simulink library "lib_dGrid"  (R2023b)
settings: Solver=VariableStepAuto  StartTime=0.0  StopTime=10.0  RelTol=1e-3
values from neighbouring files (symbols this model uses):
  C_PM = 10e-3    (= 0.01)    [my_MMC_param.m]
  Cbase = 1/Zbase/wb    (= 3.10849498226e-05)    [my_MMC_param.m]
  f0 = 50/fb    (= 1)    [my_MMC_param.m]
  Fn_filter = 1000    [my_MMC_param.m]
  Fnom = 50    [my_MMC_param.m]
  GFL_APC = 1    [Analysis_Main.m]    (also in initSimu.m; my_MMC_param.m)
  GFL_DVC = 2    [Analysis_Main.m]    (also in initSimu.m; my_MMC_param.m)
  GFM_APC = 3; (values programmed in EMT models)    [Analysis_Main.m]    (also in initSimu.m; my_MMC_param.m = 3)
  GFM_VF = 0    [my_MMC_param.m]
  Ibase = 2*Sbase/(3*Ubase)    [my_MMC_param.m]
  Idcb = Sbase/Udcb    [my_MMC_param.m]
  Ki_Iccsc = 5.15    [my_MMC_param.m]
  Ki_Ireg = CCCTRL.CC.ki    [my_MMC_param.m]
  Ki_Izscc = 100    [my_MMC_param.m]
  Ki_PLL = 1/(CCCTRL.PLL.v0*CCCTRL.PLL.T^2)    [my_MMC_param.m]
  Ki_Preg = 1.0*10    (= 10)    [my_MMC_param.m]
  Ki_Qreg = 1.0*10    (= 10)    [my_MMC_param.m]
  Ki_VAC_GFL = 50    [my_MMC_param.m]
  Ki_VACreg = 10    [my_MMC_param.m]
  Ki_VDCreg = 10    [my_MMC_param.m]
  Ki_WtReg = Kp_WtReg / 0.025    (= 1600)    [my_MMC_param.m]
  Kp_Iccsc = 0.21    [my_MMC_param.m]
  Kp_Ireg = CCCTRL.CC.kp    [my_MMC_param.m]
  Kp_Izscc = 10    [my_MMC_param.m]
  Kp_PLL = 2/CCCTRL.PLL.v0/CCCTRL.PLL.T    [my_MMC_param.m]
  Kp_Preg = 0.5/3*1    (= 0.166666666667)    [my_MMC_param.m]
  Kp_Qreg = 0.5/3*1    (= 0.166666666667)    [my_MMC_param.m]
  Kp_VAC_GFL = 0.5    [my_MMC_param.m]
  Kp_VACreg = 0.01    [my_MMC_param.m]
  Kp_VDCreg = 1    [my_MMC_param.m]
  Kp_WtReg = 40    [my_MMC_param.m]
  Kpv_GFM = 1    [my_MMC_param.m]
  Kpwm = 0.5    [my_MMC_param.m]
  Larm = Larm_pu*(Zbase/wb)    (= 0.0488923985178)    [my_MMC_param.m]
  Lff = Larm_pu/2    (= 0.075)    [my_MMC_param.m]
  Limits_Ireg = [ 2.0  -2.0]    [my_MMC_param.m]
  Limits_Preg = [ 2, -2 ]    [my_MMC_param.m]
  Limits_Qreg = 2*[ 0.42, -0.42 ]    [my_MMC_param.m]
  Limits_VACreg = [ 1.3  -1.3]    [my_MMC_param.m]
  Limits_VDCreg = [ 2.0  -2.0]    [my_MMC_param.m]
  MMC1 = MMC    [Analysis_Main.m]    (also in initSimu.m)
  Nb_PM = 400    [my_MMC_param.m]
  PhaseDelay = 1.0*Ts_Control*2*pi*50    (= 0.0628318530718)    [my_MMC_param.m]
  Pnom = 1000e6    (= 1000000000)    [my_MMC_param.m]
  Rarm = Rarm_pu*Zbase    (= 0.1536)    [my_MMC_param.m]
  Slope_Pref = 0.5    [my_MMC_param.m]
  Slope_Qref = 0.5    [my_MMC_param.m]
  Slope_Vdc_ref = Vnom_dc/2    (= 320000)    [my_MMC_param.m]
  Tdeblock = 1.5    [my_MMC_param.m]
  Ton_CROSSreg = Ton_PQreg+3    (= 7)    [my_MMC_param.m]
  Ton_PQreg = 4    [my_MMC_param.m]
  Ton_VDCreg = 1.5    [my_MMC_param.m]
  Ts = Ts_Control    (= 0.0002)    [my_MMC_param.m]
  Ts_Control = Ts_Power*2    (= 0.0002)    [my_MMC_param.m]
  Ts_Power = 20e-6 * 5    (= 0.0001)    [my_MMC_param.m]
  Ubase = sqrt(2/3)*Vnom_sec    [my_MMC_param.m]
  Udcb = 2*Ubase    [my_MMC_param.m]
  Vc0_PM = 0    [my_MMC_param.m]
  Vnom_dc = 640e3    (= 640000)    [my_MMC_param.m]
  Vnom_sec = 320e3    (= 320000)    [my_MMC_param.m]
  wb = 2*pi*fb    (= 314.159265359)    [my_MMC_param.m]
  Wt_ref_pu = 0.5 * C_PM * (Vnom_dc/Nb_PM)^2 * Nb_PM * 6 / Pnom    (= 0.03072)    [my_MMC_param.m]
undefined symbols (not defined in the file or in its folder): ControlSampleTime, DiscIntNeverNeededParam, MMC, PLL, VSM
libraries: simulink x50, spsCurrentMeasurementLib x20, spsSecondOrderFilterLib x20, spsDiodeLib x12, spsControlledVoltageSourceLib x12, spsSeriesRLCBranchLib x10, spsFirstOrderFilterLib x9, spsVoltageMeasurementLib x8, spsMeanLib x7, FriedrichLibrary x6, $bdroot x6, powerlib_extras x4
(part 4 of 8)

== system lib_dGrid/MMC-configurable control modes/MMC Control/VSM Control ==
  IdIq : Inport  PortDimensions=2
  VdVq : Inport  Port=2  PortDimensions=2
  Pref : Inport  Port=3  PortDimensions=1
  Qref : Inport  Port=4  PortDimensions=1
  wt_PLL : Inport  Port=5  PortDimensions=1
  Pmeas : Inport  Port=6
  Qmeas : Inport  Port=7
  Enable : EnablePort  StatesWhenEnabling=reset
  Add : Sum  Inputs=-++
  Bus Selector1 : BusSelector  OutputSignals=enable,Param.VSM,sp_VSM
  Constant : Constant  Value=1.12
  Constant1 : Constant  Value=[0 0]
  DQ damping1 Need New paras or New implementation : Subsystem  Commented=on  mask(Lead Lag){OmLead=VSM.VTFF.OmLead, OmLag=VSM.VTFF.OmLag}
      mask prompts: OmLead "Omega Lead"; OmLag "Omega Lag"
  Gain : Gain  Commented=on  Gain=0
  Gain4 : Gain  Gain=[1 0]
  Gain7 : Gain  Gain=Ctrl.IsVIinGFM
  Inner Loop Control : Subsystem
  Inner loop flag : Constant  Value=Ctrl.IsCCinGFM
  Modulation Gain : Subsystem  Commented=through
  Mux3 : Mux  Inputs=2
  Saturation : Saturate  Commented=through  UpperLimit=Limits_Ireg(1)  LowerLimit=Limits_Ireg(2)
  Second-Order Filter2 : spsSecondOrderFilterLib/Second-Order Filter  Commented=through  FilterType=Lowpass  Fo=Fn_filter  Zeta=Zeta_filter  Ts=Ts  Initialize=off  Vac_Init="[0,  0,  60]"  Vdc_Init=0  PlotResponse=off  FreqRange=[0, 500, 1]
      settings: LibrarySourceBlock=|
      | sps_lib/Control/Filters/Second-Order
      | Filter
  Should it be a coeffecient in the left block? : Gain  Commented=through  Gain=0.5
  Step : Step  Commented=on  Time=5  SampleTime=Ts_Control
  Switch2 : Switch  Criteria=u2 > Threshold  Threshold=0.5  SaturateOnIntegerOverflow=off  InputSameDT=off
  Unit Delay : UnitDelay  SampleTime=Ts_Control  HasFrameUpgradeWarning=on
  VSM1 : Subsystem
  Virtual circuit daniel style1 : Subsystem
  cmd_VSM : Subsystem
  Uref_dq : Outport  VectorParamsAs1DForOutWhenUnconnected=off
  Phi [rad] : Outport  Port=2  VectorParamsAs1DForOutWhenUnconnected=off
  meas_theta_GFM : Outport  Port=3  VectorParamsAs1DForOutWhenUnconnected=off
  wires:
  Should it be a coeffecient in the left block?/1 -> Saturation/1
  Modulation Gain/1(out) -> Should it be a coeffecient in the left block?/1
  VSM1/1(E [pu]) -> Gain4/1
  Gain4/1 -> Add/2
  Constant/1 -> VSM1/5(init E [pu])
  wt_PLL/1 -> VSM1/4(init Phi [rad])
  cmd_VSM/1(cmd_ac) -> Bus Selector1/1
  Bus Selector1/3 -> VSM1/2(sp_VSM)  "<sp_VSM>"
  Bus Selector1/1 -> Unit Delay/1  "<enable>"
  Bus Selector1/2 -> VSM1/1(Param)  "<VSM>"
  Unit Delay/1 -> VSM1/Enable
  Mux3/1 -> VSM1/3(PQ_meas[pu])
  Step/1 -> DQ damping1 Need New paras or New implementation/1(enable_damp_dq)
  VdVq/1 -> DQ damping1 Need New paras or New implementation/2(u_dq0), Second-Order Filter2/1
  Constant1/1 -> Add/3
  Virtual circuit daniel style1/1(v_vc_dq) -> Gain7/1
  Gain7/1 -> Add/1
  Saturation/1 -> Uref_dq/1
  IdIq/1 -> Virtual circuit daniel style1/1(i_dq), Inner Loop Control/1(IdIq)
  DQ damping1 Need New paras or New implementation/1(damp_dq0) -> Gain/1
  Second-Order Filter2/1 -> Inner Loop Control/3(VdVq)
  Inner Loop Control/1(Out) -> Switch2/1
  Add/1 -> Switch2/3, Inner Loop Control/2(In)
  Switch2/1 -> Modulation Gain/1(Uref)
  Inner loop flag/1 -> Switch2/2, Inner Loop Control/Enable
  Pmeas/1 -> Mux3/1
  Qmeas/1 -> Mux3/2
  Pref/1 -> cmd_VSM/1(Pref)  "2"
  Qref/1 -> cmd_VSM/2(Qref)  "2"
  VSM1/3(meas_theta_GFM) -> meas_theta_GFM/1
  VSM1/2(wt_VSM) -> Phi [rad]/1

== system lib_dGrid/MMC-configurable control modes/MMC Control/u//l arms to ac//dc ==
  In1 : Inport
  In2 : Inport  Port=2
  In3 : Inport  Port=3
  In4 : Inport  Port=4
  Gain2 : Gain  Gain=1/2
  I->pu (Ibase instead of Idcb) : Gain  Gain=1/Ibase  SaturateOnIntegerOverflow=on  OutDataTypeStr=Inherit: Same as input  ParamDataTypeStr=Inherit: Same as input
  Plus1 : Sum  Inputs=+-
  Plus2 : Sum
  Plus3 : Sum
  V->pu1 : Gain  Gain=Nb_PM/Ubase  SaturateOnIntegerOverflow=on  OutDataTypeStr=Inherit: Same as input  ParamDataTypeStr=Inherit: Same as input
  V->pu2 : Gain  Gain=Nb_PM/Ubase  SaturateOnIntegerOverflow=on  OutDataTypeStr=Inherit: Same as input  ParamDataTypeStr=Inherit: Same as input
  Out1 : Outport
  Out2 : Outport  Port=2
  Out3 : Outport  Port=3
  wires:
  Gain2/1 -> I->pu (Ibase instead of Idcb)/1
  Plus3/1 -> V->pu1/1
  Plus2/1 -> Gain2/1
  In2/1 -> Plus3/1, Plus1/2
  In1/1 -> Plus3/2, Plus1/1
  Plus1/1 -> V->pu2/1
  In3/1 -> Plus2/1
  I->pu (Ibase instead of Idcb)/1 -> Out3/1
  In4/1 -> Plus2/2
  V->pu1/1 -> Out1/1
  V->pu2/1 -> Out2/1

== system lib_dGrid/TL-VSC-configurable control modes/VSC Control/APC & Q//Vac Regulator ==
  note: Reactive Power Regulator
  note: Active Power Regulator
  Pmeas : Inport  PortDimensions=1
  Pref : Inport  Port=2  PortDimensions=1  SampleTime=Ts
  Qmes : Inport  Port=3  PortDimensions=1
  Qref : Inport  Port=4  PortDimensions=1
  VdVq_mes : Inport  Port=5  PortDimensions=2
  Enable : EnablePort  StatesWhenEnabling=reset
  Constant : Constant  Value=Ctrl.IsVacGFL
  Discrete-Time Integrator : DiscreteIntegrator  SampleTime=Ts  LimitOutput=on  UpperSaturationLimit=Limits_Qreg(1)  LowerSaturationLimit=Limits_Qreg(2)  ICPrevOutput=DiscIntNeverNeededParam  ICPrevScaledInput=DiscIntNeverNeededParam
  Discrete-Time Integrator1 : DiscreteIntegrator  SampleTime=Ts  LimitOutput=on  UpperSaturationLimit=Limits_Preg(1)  LowerSaturationLimit=Limits_Preg(2)  ICPrevOutput=DiscIntNeverNeededParam  ICPrevScaledInput=DiscIntNeverNeededParam
  Product{,1..3} (4 alike) : Product  RndMeth=Zero
  Rtot_pu1 : Gain  Gain=-1  SaturateOnIntegerOverflow=on  OutDataTypeStr=Inherit: Same as input  ParamDataTypeStr=Inherit: Same as input
  Saturation1 : Saturate  UpperLimit=Limits_Preg(1)  LowerLimit=Limits_Preg(2)  SampleTime=Ts
  Saturation2 : Saturate  UpperLimit=Limits_Qreg(1)  LowerLimit=Limits_Qreg(2)
  Sum : Sum  Inputs=|-+
  Sum1 : Sum  Inputs=|-+
  Sum2 : Sum  InputSameDT=on  SaturateOnIntegerOverflow=on  SampleTime=Ts  OutDataTypeStr=Inherit: Same as first input
  Sum6 : Sum  InputSameDT=on  SaturateOnIntegerOverflow=on  SampleTime=Ts  OutDataTypeStr=Inherit: Same as first input
  Switch3 : Switch  Criteria=u2 > Threshold  Threshold=0.5  OutDataTypeStr=double  SaturateOnIntegerOverflow=off  InputSameDT=off
  VAC control : Subsystem
  VdcNom_SM : Constant  Value=Kp_Qreg
  VdcNom_SM1 : Constant  Value=Ki_Qreg
  VdcNom_SM2 : Constant  Value=Kp_Preg  SampleTime=Ts
  VdcNom_SM3 : Constant  Value=Ki_Preg  SampleTime=Ts
  Zero-Order Hold : ZeroOrderHold  Commented=through  SampleTime=Ts
  Zero-Order Hold1 : ZeroOrderHold  Commented=through  SampleTime=Ts
  Id_ref_Pctrl : Outport  SampleTime=Ts  VectorParamsAs1DForOutWhenUnconnected=off
  Iq_ref : Outport  Port=2  VectorParamsAs1DForOutWhenUnconnected=off
  wires:
  Saturation2/1 -> Rtot_pu1/1
  Switch3/1 -> Iq_ref/1
  Sum6/1 -> Saturation2/1
  Sum/1 -> Product1/2, Product/2
  Product/1 -> Discrete-Time Integrator/1
  Product1/1 -> Zero-Order Hold/1
  VdcNom_SM/1 -> Product1/1
  VdcNom_SM1/1 -> Product/1
  Discrete-Time Integrator/1 -> Sum6/2
  Zero-Order Hold/1 -> Sum6/1
  Qref/1 -> Sum/2
  Rtot_pu1/1 -> Switch3/3
  Constant/1 -> Switch3/2, VAC control/Enable
  VdVq_mes/1 -> VAC control/1(Vdq_meas)
  VAC control/1(Out1) -> Switch3/1
  VdcNom_SM3/1 -> Product2/1
  Product3/1 -> Zero-Order Hold1/1
  Pmeas/1 -> Sum1/1
  Discrete-Time Integrator1/1 -> Sum2/2
  Zero-Order Hold1/1 -> Sum2/1
  Product2/1 -> Discrete-Time Integrator1/1
  Sum1/1 -> Product3/2, Product2/2
  Pref/1 -> Sum1/2
  Saturation1/1 -> Id_ref_Pctrl/1
  VdcNom_SM2/1 -> Product3/1
  Sum2/1 -> Saturation1/1
  Qmes/1 -> Sum/1

== system lib_dGrid/TL-VSC-configurable control modes/VSC Control/Classic//Cross GFL ->Id* ==
  Id_P : Inport
  PQreg_On : Inport  Port=2
  Id_Udc : Inport  Port=3
  Iq_ref : Inport  Port=4
  Mux : Mux  Inputs=2
  Switch4 : Switch  Criteria=u2 ~= 0  Threshold=0.5  OutDataTypeStr=double  SaturateOnIntegerOverflow=off  InputSameDT=off
  Out1 : Outport
  Out2 : Outport  Port=2
  wires:
  Id_P/1 -> Switch4/1
  PQreg_On/1 -> Switch4/2
  Mux/1 -> Out2/1
  Iq_ref/1 -> Mux/2
  Switch4/1 -> Mux/1, Out1/1
  Id_Udc/1 -> Switch4/3

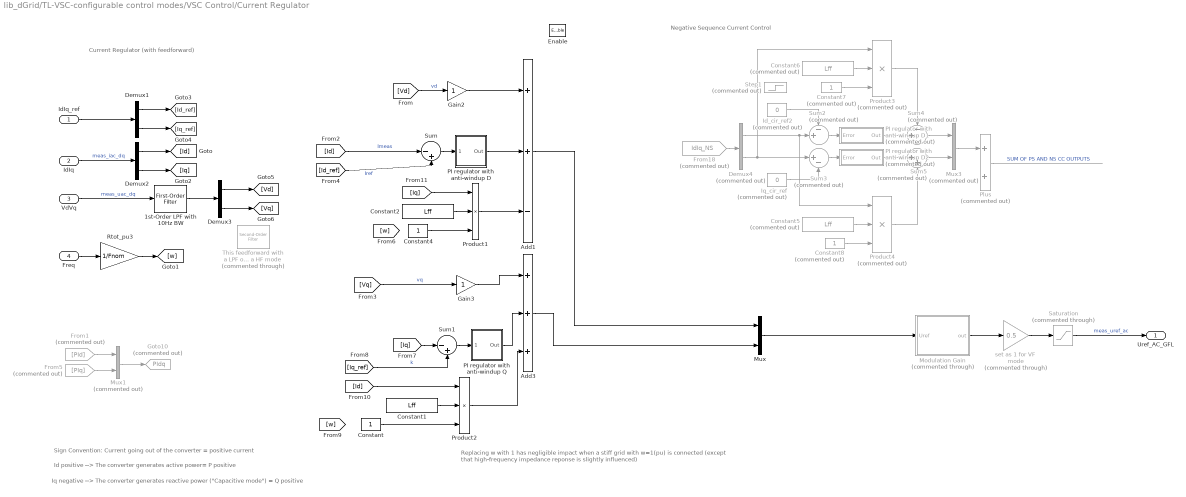
== system lib_dGrid/TL-VSC-configurable control modes/VSC Control/Current Regulator ==
  note: Negative Sequence Current Control
  note: Id positive --> The converter generates active power= P positive
  note: Iq negative --> The converter generates reactive power ("Capacitive mode") = Q positive
  note: Sign Convention: Current going out of the converter = positive current
  note: Current Regulator
      | (with feedforward)
  note: Replacing w with 1 has negligible impact
      | when a stiff grid with w=1(pu) is connected (except that high-frequency impedance reponse is slightly influenced)
  IdIq_ref : Inport  PortDimensions=2
  IdIq : Inport  Port=2  PortDimensions=2
  VdVq : Inport  Port=3  PortDimensions=2
  Freq : Inport  Port=4  PortDimensions=1
  Enable : EnablePort  StatesWhenEnabling=reset
  1st-Order LPF with 10Hz BW : spsFirstOrderFilterLib/First-Order Filter  FilterType=Lowpass  Tc=1/(2*pi*Fn_filter/100)  Ts=Ts  Initialize=off  Vac_Init=[0, 0, 50]  Vdc_Init=0  PlotResponse=off  FreqRange="[0,  200,  1]"
  Add1 : Sum  Inputs=++-
  Add3 : Sum  Inputs=+++
  Constant : Constant
  Constant1 : Constant  Value=Lff  SampleTime=Ts_Control
  Constant2 : Constant  Value=Lff  SampleTime=Ts_Control
  Constant4 : Constant
  Constant5 : Constant  Commented=on  Value=Lff  SampleTime=Ts_Control
  Constant6 : Constant  Commented=on  Value=Lff  SampleTime=Ts_Control
  Constant7 : Constant  Commented=on
  Constant8 : Constant  Commented=on
  Demux1 : Demux  Outputs=2
  Demux2 : Demux  Outputs=2
  Demux3 : Demux  Outputs=2
  Demux4 : Demux  Commented=on  Outputs=2
  From1 : From  Commented=on  GotoTag=PId
  From18 : From  Commented=on  GotoTag=IdIq_NS
  From5 : From  Commented=on  GotoTag=PIq
  Gain2 : Gain
  Gain3 : Gain
  Goto10 : Goto  Commented=on  GotoTag=PIdq  TagVisibility=global
  Id_cir_ref2 : Constant  Commented=on  Value=0
  Iq_cir_ref : Constant  Commented=on  Value=0
  Modulation Gain : Subsystem  Commented=through
  Mux : Mux  Inputs=2
  Mux1 : Mux  Commented=on  Inputs=2
  Mux3 : Mux  Commented=on  Inputs=2
  PI regulator with anti-windup D : Subsystem  DialogController=POWERSYS.PowerSysDialog  mask(Discrete PI Controller){Kp=Kp_Ireg, Ki=Ki_Ireg, Par_Limits=Limits_Ireg, Init=0, Ts=Ts}
      mask prompts: Kp "Proportional gain (Kp):"; Ki "Integral gain (Ki):"; Par_Limits "Output limits: [ Upper   Lower ]"; Init "Output initial value:"; Ts "Sample time:"
      mask help: This block implements a discrete PI controller.
      mask init:
      | UpperLimit=Par_Limits(1);
      | LowerLimit=Par_Limits(2);
      | power_initmask();
      mask Help: This block is part of a subset of blocks in the Extras library that does not have documentation associated with it, other than the block mask description.
      mask Display: disp('PI');
  PI regulator with anti-windup D1 : Subsystem  Commented=on  DialogController=POWERSYS.PowerSysDialog  mask(Discrete PI Controller){Kp=Kp_Ireg, Ki=Ki_Ireg, Par_Limits=Limits_Ireg, Init=0, Ts=Ts}
      mask prompts: Kp "Proportional gain (Kp):"; Ki "Integral gain (Ki):"; Par_Limits "Output limits: [ Upper   Lower ]"; Init "Output initial value:"; Ts "Sample time:"
      mask help: This block implements a discrete PI controller.
      mask init:
      | UpperLimit=Par_Limits(1);
      | LowerLimit=Par_Limits(2);
      | power_initmask();
      mask Help: This block is part of a subset of blocks in the Extras library that does not have documentation associated with it, other than the block mask description.
      mask Display: disp('PI');
  PI regulator with anti-windup D2 : Subsystem  Commented=on  DialogController=POWERSYS.PowerSysDialog  mask(Discrete PI Controller){Kp=Kp_Ireg, Ki=Ki_Ireg, Par_Limits=Limits_Ireg, Init=0, Ts=Ts}
      mask prompts: Kp "Proportional gain (Kp):"; Ki "Integral gain (Ki):"; Par_Limits "Output limits: [ Upper   Lower ]"; Init "Output initial value:"; Ts "Sample time:"
      mask help: This block implements a discrete PI controller.
      mask init:
      | UpperLimit=Par_Limits(1);
      | LowerLimit=Par_Limits(2);
      | power_initmask();
      mask Help: This block is part of a subset of blocks in the Extras library that does not have documentation associated with it, other than the block mask description.
      mask Display: disp('PI');
  PI regulator with anti-windup Q : Subsystem  DialogController=POWERSYS.PowerSysDialog  mask(Discrete PI Controller){Kp=Kp_Ireg, Ki=Ki_Ireg, Par_Limits=Limits_Ireg, Init=0, Ts=Ts}
      mask prompts: Kp "Proportional gain (Kp):"; Ki "Integral gain (Ki):"; Par_Limits "Output limits: [ Upper   Lower ]"; Init "Output initial value:"; Ts "Sample time:"
      mask help: This block implements a discrete PI controller.
      mask init:
      | UpperLimit=Par_Limits(1);
      | LowerLimit=Par_Limits(2);
      | power_initmask();
      mask Help: This block is part of a subset of blocks in the Extras library that does not have documentation associated with it, other than the block mask description.
      mask Display: disp('PI');
  Plus : Sum  Commented=on
  Product1 : Product  Inputs=3  RndMeth=Zero
  Product2 : Product  Inputs=3  RndMeth=Zero
  Product3 : Product  Commented=on  Inputs=3  RndMeth=Zero
  Product4 : Product  Commented=on  Inputs=3  RndMeth=Zero
  Rtot_pu3 : Gain  Gain=1/Fnom  SaturateOnIntegerOverflow=on  OutDataTypeStr=Inherit: Same as input  ParamDataTypeStr=Inherit: Same as input
  Saturation : Saturate  Commented=through  UpperLimit=Limits_Ireg(1)  LowerLimit=Limits_Ireg(2)
  Step1 : Step  Commented=on  Time=10  After=0.02  SampleTime=0
  Sum : Sum  Inputs=|-+
  Sum1 : Sum  Inputs=|-+
  Sum2 : Sum  Commented=on  Inputs=-+|
  Sum3 : Sum  Commented=on  Inputs=|+-
  Sum4 : Sum  Commented=on  Inputs=-+|
  Sum5 : Sum  Commented=on  Inputs=|++
  This feedforward with a LPF of 1kHz possibly induce a HF mode : spsSecondOrderFilterLib/Second-Order Filter  Commented=through  FilterType=Lowpass  Fo=Fn_filter  Zeta=Zeta_filter  Ts=Ts  Initialize=off  Vac_Init="[0,  0,  60]"  Vdc_Init=0  PlotResponse=off  FreqRange=[0, 500, 1]
      settings: LibrarySourceBlock=|
      | sps_lib/Control/Filters/Second-Order
      | Filter
  set as 1 for VF mode : Gain  Commented=through  Gain=0.5
  Uref_AC_GFL : Outport  VectorParamsAs1DForOutWhenUnconnected=off
  wires:
  Mux1/1 -> Goto10/1
  Saturation/1 -> Uref_AC_GFL/1  "meas_uref_ac"
  PI regulator with anti-windup D/1(Out) -> Add1/2
  PI regulator with anti-windup Q/1(Out) -> Add3/2
  [Vd] -> Gain2/1  "vd"
  Product2/1 -> Add3/3
  [Vq] -> Gain3/1  "vq"
  Demux2/1 -> [Id]
  IdIq/1 -> Demux2/1  "meas_iac_dq"
  [Id] -> Sum/1  "Imeas"
  [Iq] -> Sum1/1
  Demux2/2 -> [Iq]
  From5/1 -> Mux1/2
  From1/1 -> Mux1/1
  Constant4/1 -> Product1/3
  Constant2/1 -> Product1/2
  Constant/1 -> Product2/3
  Constant1/1 -> Product2/2
  Sum1/1 -> PI regulator with anti-windup Q/1(Error)
  Sum/1 -> PI regulator with anti-windup D/1(Error)
  VdVq/1 -> 1st-Order LPF with 10Hz BW/1  "meas_uac_dq"
  Demux3/2 -> [Vq]
  Demux3/1 -> [Vd]
  IdIq_ref/1 -> Demux1/1
  Demux1/2 -> [Iq_ref]
  Demux1/1 -> [Id_ref]
  Rtot_pu3/1 -> [w]
  Freq/1 -> Rtot_pu3/1
  Add1/1 -> Mux/1
  Add3/1 -> Mux/2
  Gain2/1 -> Add1/1
  Gain3/1 -> Add3/1
  set as 1 for VF mode/1 -> Saturation/1
  Modulation Gain/1(out) -> set as 1 for VF mode/1
  [Id] -> Product2/1
  [Iq] -> Product1/1
  Mux/1 -> Modulation Gain/1(Uref)
  1st-Order LPF with 10Hz BW/1 -> Demux3/1
  Sum5/1 -> Mux3/2
  Constant5/1 -> Product4/2
  Demux4/1 -> Product4/1, Sum2/2
  Iq_cir_ref/1 -> Sum3/2
  From18/1 -> Demux4/1
  Sum3/1 -> PI regulator with anti-windup D2/1(Error)
  Id_cir_ref2/1 -> Sum2/1
  Sum2/1 -> PI regulator with anti-windup D1/1(Error)
  PI regulator with anti-windup D1/1(Out) -> Sum4/2
  PI regulator with anti-windup D2/1(Out) -> Sum5/1
  Sum4/1 -> Mux3/1
  Product4/1 -> Sum5/2
  Constant7/1 -> Product3/3
  Constant6/1 -> Product3/2
  Demux4/2 -> Product3/1, Sum3/1
  Product3/1 -> Sum4/1
  Constant8/1 -> Product4/3
  Product1/1 -> Add1/3
  Mux3/1 -> Plus/1
  Plus/1 -> ?  "SUM OF PS AND NS CC OUTPUTS"
  [Iq_ref] -> Sum1/2  "k"
  [Id_ref] -> Sum/2  "Iref"

== system lib_dGrid/TL-VSC-configurable control modes/VSC Control/DC Voltage Regulator ** Does current direction influence the +-sign of Id_ref? ==
  note: Taking Vbase as the base voltage for dc voltage
      | Vdc_pu = Vdc_abs / Vbase = Vdc_abs / Vnom_dc * Vnom_dc / Vbase
      | small-signal control loop transfer function is
      | Id_ref = Vdc_abs / Vnom_dc * Hvdc = Vdc_abs / Vnom_dc * Vbase / Vbase * Hvdc = Vdc_pu * Vbase / Vnom_dc * Hvdc
  note: VDC Regulator
  Vdc_meas : Inport  PortDimensions=1
  Vdc_ref : Inport  Port=2  PortDimensions=1
  Enable : EnablePort  StatesWhenEnabling=reset
  "  " : Gain  Gain=-1
  1st-Order HPF : spsFirstOrderFilterLib/First-Order Filter  Commented=through  FilterType=Highpass  Tc=1/(2*pi*20)  Ts=Ts_Control  Initialize=on  Vac_Init=[0, 0, 50]  Vdc_Init=0  PlotResponse=off  FreqRange="[0,  200,  1]"
  2nd-Order LPF : spsSecondOrderFilterLib/Second-Order Filter  Commented=through  FilterType=Lowpass  Fo=Fn_filter/50  Zeta=Zeta_filter  Ts=Ts  Initialize=off  Vac_Init="[0,  0,  60]"  Vdc_Init=0  PlotResponse=off  FreqRange=[0, 500, 1]
      settings: LibrarySourceBlock=|
      | sps_lib/Control/Filters/Second-Order
      | Filter
  Constant : Constant  Commented=on  Value=Vnom_dc*0.9
  Discrete-Time Integrator : DiscreteIntegrator  SampleTime=Ts  LimitOutput=on  UpperSaturationLimit=Limits_VDCreg(1)  LowerSaturationLimit=Limits_VDCreg(2)  ICPrevOutput=DiscIntNeverNeededParam  ICPrevScaledInput=DiscIntNeverNeededParam
  Product : Product  RndMeth=Zero
  Product1 : Product  RndMeth=Zero
  Rtot_pu2 : Gain  Gain=1/Vnom_dc  SaturateOnIntegerOverflow=on  OutDataTypeStr=Inherit: Same as input  ParamDataTypeStr=Inherit: Same as input
  Saturation2 : Saturate  UpperLimit=Limits_VDCreg(1)  LowerLimit=Limits_VDCreg(2)  SampleTime=Ts
  Step : Step  Commented=on  Time=6  SampleTime=0
  Sum : Sum  Inputs=|-+
  Sum6 : Sum  InputSameDT=on  SaturateOnIntegerOverflow=on  SampleTime=Ts  OutDataTypeStr=Inherit: Same as first input
  Switch : Switch  Commented=on  Criteria=u2 > Threshold  SaturateOnIntegerOverflow=off  InputSameDT=off
  VdcNom_SM : Constant  Value=Kp_VDCreg
  VdcNom_SM1 : Constant  Value=Ki_VDCreg
  Zero-Order Hold - Negligible dynamic effect : ZeroOrderHold  Commented=through  SampleTime=Ts
  Id_ref : Outport  VectorParamsAs1DForOutWhenUnconnected=off
  wires:
  Saturation2/1 -> "  "/1
  VdcNom_SM/1 -> Product1/1
  Product/1 -> Discrete-Time Integrator/1
  Product1/1 -> Zero-Order Hold - Negligible dynamic effect/1
  VdcNom_SM1/1 -> Product/1
  Sum6/1 -> Saturation2/1
  Zero-Order Hold - Negligible dynamic effect/1 -> Sum6/1
  Vdc_ref/1 -> Sum/2
  Sum/1 -> Rtot_pu2/1
  Vdc_meas/1 -> 1st-Order HPF/1
  Rtot_pu2/1 -> Product/2, Product1/2
  "  "/1 -> Id_ref/1
  Step/1 -> Switch/2
  Constant/1 -> Switch/1
  Discrete-Time Integrator/1 -> Sum6/2
  1st-Order HPF/1 -> Sum/1

== system lib_dGrid/TL-VSC-configurable control modes/VSC Control/GFL//GFM Switching & Modulation (UCM // DM) & dq0 ->abc ==
  note: VSC CTRL MODE involving current control:
      | >2 for GFM, <0 for VF, otherwise for GFL
  note: proved with negligile effect
  note: Kpwm=0.5 can be considered to be extracted from m_ac to yield new m_ac, leading to the transformation from sum-diff to upper-lower arms as:
      | m_ac = (ml - mu)
      | m_dc = mu + ml =>
      | mu = (-m_ac + m_dc)/2
      | ml = (m_ac + m_dc)/2
  Uac_VF : Inport
  Uac_GFM : Inport  Port=2
  Uac_GFL : Inport  Port=3
  ACreg_On : Inport  Port=4
  wt_GFM : Inport  Port=5
  wt_PLL : Inport  Port=6
  wt_VF : Inport  Port=7
  " " : Subsystem
  >0 for in1 : Switch  Criteria=u2 > Threshold  SaturateOnIntegerOverflow=off  InputSameDT=off
  >2 for in1 : Switch  Criteria=u2 > Threshold  Threshold=2  SaturateOnIntegerOverflow=off  InputSameDT=off
  Constant1 : Constant  Value=CtrlMode
  Constant3 : Constant  Value=0  SampleTime=Ts
  Direct Modulation : $bdroot/MMC/MMC Control/Current Regulator/Modulation Gain  SystemSampleTime=-1  VariantActivationTime=update diagram  AllowFlexibleInterface=on  Latency=0  AutoFrameSizeCalculation=off
      link override ->pu: Gain=1/Udcb
  Gain : Gain  Gain=Kpwm
  Mux2 : Mux  Inputs=[2 1]
  Saturation : Saturate  UpperLimit=Limits_Ireg(1)  LowerLimit=Limits_Ireg(2)
  Switch2 : Switch  Criteria=u2 ~= 0  Threshold=0.5  OutDataTypeStr=double  SaturateOnIntegerOverflow=off  InputSameDT=off
  Switch3 : Switch  Criteria=u2 > Threshold  Threshold=2  SaturateOnIntegerOverflow=off  InputSameDT=off
  dq0 to abc ++ Select Alignment 2 with no phase delay : spsdq0toabcLib/dq0 to abc  Commented=on  Alignment=Aligned with phase A axis
  dq0->ab0 phi ua=cos(phi)*ud-sin(phi)*uq ub=-sin(phi)*ud+cos(phi)*uq : Subsystem  AncestorBlock=FriedrichLibrary/Transformations/dq0->ab0 phi
      mask Display:
      | plot([0 1], [0,1])
      | text(0.05,0.8,'dq0','texmode','on')
      | text(1, 0.5,'\alpha\beta0','HorizontalAlignment','right','texmode','on')
      | text(0.05,0.3,'\phi','texmode','on')
  in2>0 for in1 : Switch  Criteria=u2 > Threshold  SaturateOnIntegerOverflow=off  InputSameDT=off
  refer to TL-VSC control : Bias  Bias=PhaseDelay  SaturateOnIntegerOverflow=off
  ~=0 for in1 : Switch  Criteria=u2 ~= 0  Threshold=0.5  OutDataTypeStr=double  SaturateOnIntegerOverflow=off  InputSameDT=off
  Uref_AC : Outport
  wt : Outport  Port=2
  uac_ref_dq : Outport  Port=3
  wires:
  Uac_GFL/1 -> ~=0 for in1/3, >2 for in1/3  "Uac_ref_GFL"
  >2 for in1/1 -> >0 for in1/1
  Uac_GFM/1 -> >2 for in1/1  "Uac_ref_GFM"
  Switch3/1 -> in2>0 for in1/1
  wt_GFM/1 -> Switch3/1  "wt_GFM"
  Constant1/1 -> in2>0 for in1/2, Switch3/2, >2 for in1/2, >0 for in1/2
  ACreg_On/1 -> ~=0 for in1/2, Switch2/2
  wt_PLL/1 -> Switch2/3, Switch3/3  "wt_PLL"
  Uac_VF/1 -> >0 for in1/3  "Uac_ref_VF"
  >0 for in1/1 -> ~=0 for in1/1
  wt_VF/1 -> in2>0 for in1/3  "wt_VF"
  in2>0 for in1/1 -> Switch2/1
  refer to TL-VSC control/1 -> dq0->ab0 phi ua=cos(phi)*ud-sin(phi)*uq ub=-sin(phi)*ud+cos(phi)*uq/2(phi)
  dq0->ab0 phi ua=cos(phi)*ud-sin(phi)*uq ub=-sin(phi)*ud+cos(phi)*uq/1("ab0 ") -> " "/1(AB0)
  Switch2/1 -> refer to TL-VSC control/1, wt/1  "wt_out"
  Constant3/1 -> Mux2/2
  Saturation/1 -> uac_ref_dq/1, Mux2/1  "uac_ref_dq"
  Mux2/1 -> dq0->ab0 phi ua=cos(phi)*ud-sin(phi)*uq ub=-sin(phi)*ud+cos(phi)*uq/1(dq0)
  " "/1(abc) -> Uref_AC/1
  Direct Modulation/1 -> Gain/1
  ~=0 for in1/1 -> Direct Modulation/1  "uac_ref_dq"
  Gain/1 -> Saturation/1

== system lib_dGrid/TL-VSC-configurable control modes/VSC Control/PLL, Measurements and Transformation ==
  note: FILTER Setting for Consideration:
      | Only apply LPF to the P&Q measurements of GFL control, not to VSM control scheme (as it is not filter based), and not to the voltage and current measurements of GFL control. The bandwidth can be set as 100 Hz.
      | --- For the LPF-settings with up to 1kHz cutoff frequency, the dynamic effect could be neglected for the 0.1-300 Hz frequency range
  note: Original PQ measurement method
  note: P (pu) = Vd*Id + Vq*Iq
  note: Q (pu) = Vq*Id - Vd*Iq
  note: P positive = Converter generates active power (Inverter Mode)
  note: Q positive = Converter generates reactive power (Capacitive Mode)
  Vabc : Inport  PortDimensions=3
  Iabc : Inport  Port=2  PortDimensions=3
  wt : Inport  Port=3  PortDimensions=1
  2nd-Order LPF 100 Hz : spsSecondOrderFilterLib/Second-Order Filter  FilterType=Lowpass  Fo=Fn_filter/10  Zeta=Zeta_filter  Ts=Ts  Initialize=off  Vac_Init="[0,  0,  60]"  Vdc_Init=0  PlotResponse=off  FreqRange=[0, 500, 1]
      settings: LibrarySourceBlock=|
      | sps_lib/Control/Filters/Second-Order
      | Filter
  "2nd-Order LPF 20Hz -- BETTER NOT USE LPF for VSM synchronization" : spsSecondOrderFilterLib/Second-Order Filter  Commented=through  FilterType=Lowpass  Fo=Fn_filter/50  Zeta=Zeta_filter  Ts=Ts  Initialize=off  Vac_Init="[0,  0,  60]"  Vdc_Init=0  PlotResponse=off  FreqRange=[0, 500, 1]
      settings: LibrarySourceBlock=|
      | sps_lib/Control/Filters/Second-Order
      | Filter
  Add : Sum  Inputs=1
  Demux : Demux  Outputs=2
  Discrete Mean value : powerlib_extras/Discrete Measurements/Discrete  Mean value  Commented=through  Freq=Fnom  Vinit=0  Ts=Ts
  Discrete Mean value1 : powerlib_extras/Discrete Measurements/Discrete  Mean value  Commented=through  Freq=Fnom  Vinit=0  Ts=Ts
  Gain1 : Gain  Commented=on  Gain=-1
  I->pu2 : Gain  Gain=sqrt(3)*Vnom_sec/sqrt(2)/Pnom  SaturateOnIntegerOverflow=on  OutDataTypeStr=Inherit: Same as input  ParamDataTypeStr=Inherit: Same as input
  PhN->ab1 : Subsystem  AncestorBlock=FriedrichLibrary/Transformations/PhN->ab0
      mask Display:
      | plot([0 1], [0,1])
      | plot([0.1 0.25 0.4 0.25 0.25], [0.5 0.6 0.5 0.6 0.8]) % Stern
      | text(0.05,1,'PhN','VerticalAlignment','Top')
      | text(0.55, 0.3,'\alpha\beta0','texmode','on')
  PhN->ab2 : Subsystem  AncestorBlock=FriedrichLibrary/Transformations/PhN->ab0
      mask Display:
      | plot([0 1], [0,1])
      | plot([0.1 0.25 0.4 0.25 0.25], [0.5 0.6 0.5 0.6 0.8]) % Stern
      | text(0.05,1,'PhN','VerticalAlignment','Top')
      | text(0.55, 0.3,'\alpha\beta0','texmode','on')
  Product : Product  RndMeth=Zero
  Product1 : Product  RndMeth=Zero
  Second-Order Filter1 : spsSecondOrderFilterLib/Second-Order Filter  Commented=through  FilterType=Lowpass  Fo=Fn_filter  Zeta=Zeta_filter  Ts=Ts  Initialize=off  Vac_Init="[0,  0,  60]"  Vdc_Init=0  PlotResponse=off  FreqRange=[0, 500, 1]
      settings: LibrarySourceBlock=|
      | sps_lib/Control/Filters/Second-Order
      | Filter
  Second-Order Filter2 : spsSecondOrderFilterLib/Second-Order Filter  Commented=through  FilterType=Lowpass  Fo=Fn_filter  Zeta=Zeta_filter  Ts=Ts  Initialize=off  Vac_Init="[0,  0,  60]"  Vdc_Init=0  PlotResponse=off  FreqRange=[0, 500, 1]
      settings: LibrarySourceBlock=|
      | sps_lib/Control/Filters/Second-Order
      | Filter
  Second-Order Filter3 : spsSecondOrderFilterLib/Second-Order Filter  Commented=on  FilterType=Lowpass  Fo=Fn_filter  Zeta=Zeta_filter  Ts=Ts  Initialize=off  Vac_Init="[0,  0,  60]"  Vdc_Init=0  PlotResponse=off  FreqRange=[0, 500, 1]
      settings: LibrarySourceBlock=|
      | sps_lib/Control/Filters/Second-Order
      | Filter
  Selector1 : Selector  Commented=on  InputPortWidth=3  IndexOptions=Index vector (dialog)  Indices=[1 2]  OutputSizes=1
  Selector3 : Selector  InputPortWidth=2  IndexOptions=Index vector (dialog)  Indices=[2 1]  OutputSizes=1
  Selector4 : Selector  InputPortWidth=3  IndexOptions=Index vector (dialog)  Indices=[1 2]  OutputSizes=1
  Selector5 : Selector  InputPortWidth=3  IndexOptions=Index vector (dialog)  Indices=[1 2]  OutputSizes=1
  Subtract : Sum  Inputs=+-
  Symmetrical PLL : Subsystem  AncestorBlock=FriedrichLibrary/Discrete Stuff/Symmetrical PLL  mask{Kp_PLL=Kp_PLL, Ki_PLL=Ki_PLL, Kd_PLL=0, Ts=Ts_Control}
      mask prompts: Kp_PLL "Proportional Gain PLL"; Ki_PLL "Integral Gain PLL"; Kd_PLL "Differential Gain PLL"; Ts "SampleTime"
      mask DialogControl DescGroupVar Prompt: SRF PLL
      mask DialogControl DescTextVar Prompt: Discrete implementation of a synchronous reference phase locked loop.
  Used for NS current control : Goto  Commented=on  GotoTag=IdIq_NS  TagVisibility=global
  V->pu1 : Gain  Gain=1/(Vnom_sec/sqrt(3)*sqrt(2))  SaturateOnIntegerOverflow=on  OutDataTypeStr=Inherit: Same as input  ParamDataTypeStr=Inherit: Same as input
  ab0->dq0-NS : FriedrichLibrary/Transformations/ab0->dq0-faster  Commented=on  SystemSampleTime=-1  VariantActivationTime=update diagram  AllowFlexibleInterface=on  Latency=0  AutoFrameSizeCalculation=off
  ab0->dq0-faster : Subsystem  AncestorBlock=FriedrichLibrary/Transformations/ab0->dq0-faster
      mask Display:
      | plot([0 1], [0,1])
      | text(0.05,0.8,'\alpha\beta0','texmode','on')
      | text(1, 0.5,'dq0','HorizontalAlignment','right')
      | text(0.05,0.3,'\phi','texmode','on')
  ab0->dq0-faster1 : Subsystem  AncestorBlock=FriedrichLibrary/Transformations/ab0->dq0-faster
      mask Display:
      | plot([0 1], [0,1])
      | text(0.05,0.8,'\alpha\beta0','texmode','on')
      | text(1, 0.5,'dq0','HorizontalAlignment','right')
      | text(0.05,0.3,'\phi','texmode','on')
  abc to dq0 : spsabctodq0Lib/abc to dq0  Commented=on  Alignment=Aligned with phase A axis
  Freq : Outport  VectorParamsAs1DForOutWhenUnconnected=off
  wt_PLL : Outport  Port=2  VectorParamsAs1DForOutWhenUnconnected=off
  VdVq : Outport  Port=3  VectorParamsAs1DForOutWhenUnconnected=off
  IdIq : Outport  Port=4  VectorParamsAs1DForOutWhenUnconnected=off
  P : Outport  Port=5  VectorParamsAs1DForOutWhenUnconnected=off
  Q : Outport  Port=6  VectorParamsAs1DForOutWhenUnconnected=off
  meas_theta_ref : Outport  Port=7  VectorParamsAs1DForOutWhenUnconnected=off
  wires:
  Selector3/1 -> Product1/1
  Selector4/1 -> Product/1, Selector3/1, VdVq/1, Second-Order Filter2/1  "meas_uac_dq"
  Selector5/1 -> IdIq/1, Second-Order Filter1/1, Product1/2, Product/2  "meas_iac_dq"
  Product/1 -> Add/1
  Product1/1 -> Demux/1
  Demux/1 -> Subtract/1
  Demux/2 -> Subtract/2
  Add/1 -> Discrete Mean value/1
  Subtract/1 -> Discrete Mean value1/1
  ab0->dq0-faster/1(dq0) -> Selector4/1
  Vabc/1 -> V->pu1/1
  Iabc/1 -> I->pu2/1
  ab0->dq0-faster1/1(dq0) -> Selector5/1
  Symmetrical PLL/2(phi) -> wt_PLL/1  "wt_PLL"
  Symmetrical PLL/1(f) -> Freq/1  "f"
  PhN->ab1/1(ab0) -> ab0->dq0-faster/1(ab0)
  I->pu2/1 -> PhN->ab2/1(PhN)
  PhN->ab2/1(ab0) -> Gain1/1, ab0->dq0-faster1/1(ab0)
  "2nd-Order LPF 20Hz -- BETTER NOT USE LPF for VSM synchronization"/1 -> P/1
  2nd-Order LPF 100 Hz/1 -> Q/1
  wt/1 -> ab0->dq0-faster/2(w), ab0->dq0-faster1/2(w), ab0->dq0-NS/2  "wt"
  V->pu1/1 -> PhN->ab1/1(PhN), Symmetrical PLL/1(Vabc_PhN)
  Discrete Mean value/1 -> "2nd-Order LPF 20Hz -- BETTER NOT USE LPF for VSM synchronization"/1
  Discrete Mean value1/1 -> 2nd-Order LPF 100 Hz/1
  Gain1/1 -> ab0->dq0-NS/1
  ab0->dq0-NS/1 -> Selector1/1
  Selector1/1 -> Second-Order Filter3/1  "meas_iac_dq_NS"
  Second-Order Filter3/1 -> Used for NS current control/1
  Symmetrical PLL/3(meas_theta_ref) -> meas_theta_ref/1

== system lib_dGrid/TL-VSC-configurable control modes/VSC Control/PWM ==
  note: Modulation
      | Compensation
  note: - use Udc0 for mode 1
      | - use udc for mode 3 ?
      | - mode 2 is normally not used
  note: Idcb and Udcb are not used in control anymore!
      | Instead Unified AC base is applied to all AC/DC quantities.
  note: Compensated modulation
      | ** For the test setting with quasi-ideal DC voltage source, the influence on ac side impedance response is negligible
  Uref_AC : Inport  PortDimensions=3
  Vdc_meas : Inport  Port=2
  " (Hz)2" : Constant  Value=Vnom_dc  SampleTime=Ts
  ->pu1 : Gain  Gain=1/Udcb
  Avoid division by zero2 : Saturate  UpperLimit=Vnom_dc*1.25  LowerLimit=Vnom_dc*0.75
  Constant11 : Constant  Value=Ctrl.Modulation
  Divide2 : Product  Inputs=*/
  Multiport Switch : MultiPortSwitch  SaturateOnIntegerOverflow=off
  PWM Generator (2-Level) : spsPWMGenerator2LevelLib/PWM Generator (2-Level)  ModulatorType=Three-phase bridge (6 pulses)  ModulatorMode=Unsynchronized  Fc=27*50  Pc=90  nF=27  MinMax="[ -1  1 ]"  SamplingTechnique=Natural  ModulatingSignals=off  m=0.8  Freq=60  Phase=0  Ts=Ts_Power  ShowCarrierOutport=off
  Saturation1 : Saturate  UpperLimit=1.2  LowerLimit=-1.2
  Unit Delay : UnitDelay  SampleTime=Ts_Control  HasFrameUpgradeWarning=on
  m_Ctrl : Outport  VectorParamsAs1DForOutWhenUnconnected=off
  wires:
  Constant11/1 -> Multiport Switch/1
  Divide2/1 -> Saturation1/1  "m"
  Multiport Switch/1 -> Avoid division by zero2/1
  " (Hz)2"/1 -> Multiport Switch/2
  PWM Generator (2-Level)/1 -> m_Ctrl/1
  Vdc_meas/1 -> Multiport Switch/4, Multiport Switch/3  "2"
  Unit Delay/1 -> PWM Generator (2-Level)/1
  Saturation1/1 -> Unit Delay/1
  ->pu1/1 -> Divide2/2  "udc_pu"
  Avoid division by zero2/1 -> ->pu1/1
  Uref_AC/1 -> Divide2/1

== system lib_dGrid/TL-VSC-configurable control modes/VSC Control/VF mode ==
  note: AC Voltage Control
  Udq_meas : Inport
  On : Inport  Port=2  PortDimensions=1
  IdIq : Inport  Port=3
  Enable : EnablePort  StatesWhenEnabling=reset
  Add1 : Sum  Commented=on  Inputs=+-
  Constant1 : Constant  Value=50
  Constant2 : Constant  Commented=on  Value=2*pi*f0*50
  Constant9 : Constant  Value=2*pi
  Demux1 : Demux  Outputs=2
  Demux2 : Demux  Outputs=2
  Discrete-Time Integrator : DiscreteIntegrator  InitialCondition=0*pi/180  SampleTime=Ts  ICPrevOutput=DiscIntNeverNeededParam  ICPrevScaledInput=DiscIntNeverNeededParam
  For VF mode : Math  Operator=mod  SignedPower=on
  Gain : Gain  Gain=Lff*0
  Gain1 : Gain  Gain=Lff*0
  Gain2 : Gain  Gain=2*pi
  Integrator (discrete)1 : DiscreteIntegrator  Commented=on  IntegratorMethod=Integration: Backward Euler  gainval=1  SampleTime=Ts_Control  ICPrevOutput=DiscIntNeverNeededParam  ICPrevScaledInput=DiscIntNeverNeededParam
  Mux4 : Mux  Inputs=2
  PI regulator with anti-windup D1 : Subsystem  DialogController=POWERSYS.PowerSysDialog  mask(Discrete PI Controller){Kp=Kp_VACreg, Ki=Ki_VACreg, Par_Limits=Limits_VACreg, Init=0, Ts=Ts}
      mask prompts: Kp "Proportional gain (Kp):"; Ki "Integral gain (Ki):"; Par_Limits "Output limits: [ Upper   Lower ]"; Init "Output initial value:"; Ts "Sample time:"
      mask help: This block implements a discrete PI controller.
      mask init:
      | UpperLimit=Par_Limits(1);
      | LowerLimit=Par_Limits(2);
      | power_initmask();
      mask Help: This block is part of a subset of blocks in the Extras library that does not have documentation associated with it, other than the block mask description.
      mask Display: disp('PI');
  PI regulator with anti-windup D2 : Subsystem  DialogController=POWERSYS.PowerSysDialog  mask(Discrete PI Controller){Kp=Kp_VACreg, Ki=Ki_VACreg, Par_Limits=Limits_VACreg, Init=0, Ts=Ts}
      mask prompts: Kp "Proportional gain (Kp):"; Ki "Integral gain (Ki):"; Par_Limits "Output limits: [ Upper   Lower ]"; Init "Output initial value:"; Ts "Sample time:"
      mask help: This block implements a discrete PI controller.
      mask init:
      | UpperLimit=Par_Limits(1);
      | LowerLimit=Par_Limits(2);
      | power_initmask();
      mask Help: This block is part of a subset of blocks in the Extras library that does not have documentation associated with it, other than the block mask description.
      mask Display: disp('PI');
  Saturation : Saturate  Commented=through  UpperLimit=1.3  LowerLimit=-1.3
  Should be 0 : Display  Commented=on
  Sum4 : Sum  Inputs=+-|
  Sum5 : Sum  Inputs=|-+
  Sum6 : Sum  Inputs=++|
  Sum7 : Sum  Inputs=|+-
  Switch1 : Switch  Criteria=u2 ~= 0  Threshold=0.5  OutDataTypeStr=double  SaturateOnIntegerOverflow=off  InputSameDT=off
  Ud_ref : Constant
  Udq_ref : Constant  Value=[1 0]
  Uq_ref : Constant  Value=0
  Uref_AC : Outport  VectorParamsAs1DForOutWhenUnconnected=off
  wt_VF : Outport  Port=2  VectorParamsAs1DForOutWhenUnconnected=off
  wires:
  Saturation/1 -> Uref_AC/1
  Mux4/1 -> Saturation/1
  For VF mode/1 -> wt_VF/1  "wt"
  Discrete-Time Integrator/1 -> For VF mode/1
  Constant1/1 -> Gain2/1  "f"
  Constant9/1 -> For VF mode/2
  Switch1/1 -> Demux1/1  "Umeas"
  Demux1/2 -> Sum5/1  "Uq_meas"
  Ud_ref/1 -> Sum4/1
  Demux1/1 -> Sum4/2  "Ud_meas"
  Uq_ref/1 -> Sum5/2
  Udq_meas/1 -> Switch1/1
  On/1 -> Switch1/2
  Udq_ref/1 -> Switch1/3  "Uref"
  Gain1/1 -> Sum7/2
  Gain/1 -> Sum6/1
  Sum4/1 -> PI regulator with anti-windup D1/1(Error)
  Sum6/1 -> Mux4/1
  PI regulator with anti-windup D2/1(Out) -> Sum7/1
  Sum7/1 -> Mux4/2
  PI regulator with anti-windup D1/1(Out) -> Sum6/2
  Sum5/1 -> PI regulator with anti-windup D2/1(Error)
  Gain2/1 -> Add1/1, Discrete-Time Integrator/1
  Constant2/1 -> Add1/2
  Add1/1 -> Integrator (discrete)1/1  "d_w"
  Integrator (discrete)1/1 -> Should be 0/1  "meas_theta_VF"
  Demux2/2 -> [Iq]
  IdIq/1 -> Demux2/1  "meas_iac_dq"
  Demux2/1 -> [Id]
  [Iq] -> Gain/1  "Imeas"
  [Id] -> Gain1/1  "Imeas"

== system lib_dGrid/TL-VSC-configurable control modes/VSC Control/VSM Control ==
  IdIq : Inport  PortDimensions=2
  VdVq : Inport  Port=2  PortDimensions=2
  Pref : Inport  Port=3  PortDimensions=1
  Qref : Inport  Port=4  PortDimensions=1
  wt_PLL : Inport  Port=5  PortDimensions=1
  Pmeas : Inport  Port=6
  Qmeas : Inport  Port=7
  Enable : EnablePort  StatesWhenEnabling=reset
  Add : Sum  Inputs=-++
  Bus Selector1 : BusSelector  OutputSignals=enable,Param.VSM,sp_VSM
  Constant : Constant  Value=1.12
  Constant1 : Constant  Value=[0 0]
  DQ damping1 Need New paras or New implementation : Subsystem  Commented=on  mask(Lead Lag){OmLead=VSM.VTFF.OmLead, OmLag=VSM.VTFF.OmLag}
      mask prompts: OmLead "Omega Lead"; OmLag "Omega Lag"
  Gain : Gain  Commented=on  Gain=0
  Gain4 : Gain  Gain=[1 0]
  Gain7 : Gain  Gain=Ctrl.IsVIinGFM
  Inner Loop Control : Subsystem
  Inner loop flag : Constant  Value=Ctrl.IsCCinGFM
  Modulation Gain : Subsystem  Commented=through
  Mux3 : Mux  Inputs=2
  Saturation : Saturate  Commented=through  UpperLimit=Limits_Ireg(1)  LowerLimit=Limits_Ireg(2)
  Second-Order Filter2 : spsSecondOrderFilterLib/Second-Order Filter  Commented=through  FilterType=Lowpass  Fo=Fn_filter  Zeta=Zeta_filter  Ts=Ts  Initialize=off  Vac_Init="[0,  0,  60]"  Vdc_Init=0  PlotResponse=off  FreqRange=[0, 500, 1]
      settings: LibrarySourceBlock=|
      | sps_lib/Control/Filters/Second-Order
      | Filter
  Should it be a coeffecient in the left block? : Gain  Commented=through  Gain=0.5
  Step : Step  Commented=on  Time=5  SampleTime=Ts_Control
  Switch2 : Switch  Criteria=u2 > Threshold  Threshold=0.5  SaturateOnIntegerOverflow=off  InputSameDT=off
  Unit Delay : UnitDelay  SampleTime=Ts_Control  HasFrameUpgradeWarning=on
  VSM1 : Subsystem
  Virtual circuit daniel style1 : Subsystem
  cmd_VSM : Subsystem
  Uref_dq : Outport  VectorParamsAs1DForOutWhenUnconnected=off
  Phi [rad] : Outport  Port=2  VectorParamsAs1DForOutWhenUnconnected=off
  meas_theta_GFM : Outport  Port=3  VectorParamsAs1DForOutWhenUnconnected=off
  wires:
  Should it be a coeffecient in the left block?/1 -> Saturation/1
  Modulation Gain/1(out) -> Should it be a coeffecient in the left block?/1
  VSM1/1(E [pu]) -> Gain4/1
  Gain4/1 -> Add/2
  Constant/1 -> VSM1/5(init E [pu])
  wt_PLL/1 -> VSM1/4(init Phi [rad])
  cmd_VSM/1(cmd_ac) -> Bus Selector1/1
  Bus Selector1/3 -> VSM1/2(sp_VSM)  "<sp_VSM>"
  Bus Selector1/1 -> Unit Delay/1  "<enable>"
  Bus Selector1/2 -> VSM1/1(Param)  "<VSM>"
  Unit Delay/1 -> VSM1/Enable
  Mux3/1 -> VSM1/3(PQ_meas[pu])
  Step/1 -> DQ damping1 Need New paras or New implementation/1(enable_damp_dq)
  VdVq/1 -> DQ damping1 Need New paras or New implementation/2(u_dq0), Second-Order Filter2/1
  Constant1/1 -> Add/3
  Virtual circuit daniel style1/1(v_vc_dq) -> Gain7/1
  Gain7/1 -> Add/1
  Saturation/1 -> Uref_dq/1
  IdIq/1 -> Virtual circuit daniel style1/1(i_dq), Inner Loop Control/1(IdIq)
  DQ damping1 Need New paras or New implementation/1(damp_dq0) -> Gain/1
  Second-Order Filter2/1 -> Inner Loop Control/3(VdVq)
  Inner Loop Control/1(Out) -> Switch2/1
  Add/1 -> Switch2/3, Inner Loop Control/2(In)
  Switch2/1 -> Modulation Gain/1(Uref)
  Inner loop flag/1 -> Switch2/2, Inner Loop Control/Enable
  Pmeas/1 -> Mux3/1
  Qmeas/1 -> Mux3/2
  Pref/1 -> cmd_VSM/1(Pref)  "2"
  Qref/1 -> cmd_VSM/2(Qref)  "2"
  VSM1/3(meas_theta_GFM) -> meas_theta_GFM/1
  VSM1/2(wt_VSM) -> Phi [rad]/1

== system lib_dGrid/MMC-configurable control modes/MMC Control/APC & Q//Vac Regulator/VAC control ==
  Vdq_meas : Inport
  Enable : EnablePort  StatesWhenEnabling=reset
  1st-Order LPF : spsFirstOrderFilterLib/First-Order Filter  FilterType=Lowpass  Tc=1/(2*pi*Fn_filter/100)  Ts=Ts  Initialize=on  Vac_Init=[0, 0, 50]  Vdc_Init=0  PlotResponse=off  FreqRange="[0,  200,  1]"
  Abs : Abs  SaturateOnIntegerOverflow=off
  Demux : Demux  Outputs=2
  Discrete-Time Integrator1 : DiscreteIntegrator  SampleTime=Ts  LimitOutput=on  UpperSaturationLimit=1.5  LowerSaturationLimit=-1.5  ICPrevOutput=DiscIntNeverNeededParam  ICPrevScaledInput=DiscIntNeverNeededParam
  Product2 : Product  RndMeth=Zero
  Product3 : Product  RndMeth=Zero
  Real-Imag to Complex : RealImagToComplex
  Rtot_pu2 : Gain  Gain=-1  SaturateOnIntegerOverflow=on  OutDataTypeStr=Inherit: Same as input  ParamDataTypeStr=Inherit: Same as input
  Saturation3 : Saturate  UpperLimit=1  LowerLimit=-1
  Scope1 : Scope  Commented=on  NumInputPorts=2
  Sum1 : Sum  Inputs=|-+
  Sum2 : Sum  InputSameDT=on  SaturateOnIntegerOverflow=on  SampleTime=Ts  OutDataTypeStr=Inherit: Same as first input
  VdcNom_SM2 : Constant  Value=Kp_VAC_GFL
  VdcNom_SM3 : Constant  Value=Ki_VAC_GFL
  Vref : Constant
  Vref_Tstep : Step  Commented=on  Time=5  Before=1  After=1.03  SampleTime=0
  Zero-Order Hold1 : ZeroOrderHold  Commented=through  SampleTime=Ts
  Out1 : Outport
  wires:
  Abs/1 -> Sum1/1
  Discrete-Time Integrator1/1 -> Sum2/2
  Saturation3/1 -> Rtot_pu2/1
  Product3/1 -> Zero-Order Hold1/1
  Sum1/1 -> Product3/2, Product2/2
  Real-Imag to Complex/1 -> Abs/1
  VdcNom_SM2/1 -> Product3/1
  Demux/1 -> Real-Imag to Complex/1
  Demux/2 -> Real-Imag to Complex/2
  VdcNom_SM3/1 -> Product2/1
  Zero-Order Hold1/1 -> Sum2/1
  Product2/1 -> Discrete-Time Integrator1/1
  Vdq_meas/1 -> 1st-Order LPF/1
  Vref/1 -> Scope1/1, Sum1/2
  Sum2/1 -> Saturation3/1
  1st-Order LPF/1 -> Demux/1
  Rtot_pu2/1 -> Out1/1

== system lib_dGrid/MMC-configurable control modes/MMC Control/CCSC + ZSCC control/  ==
  AB0 : Inport
  Gain : Gain  Gain=1/2
  ab0->abc : Gain  Gain=[2 0 2; -1 sqrt(3) 2; -1 -sqrt(3) 2]  Multiplication=Matrix(K*u) (u vector)
  abc : Outport  SampleTime=Ts_Control  VectorParamsAs1DForOutWhenUnconnected=off
  wires:
  ab0->abc/1 -> abc/1
  AB0/1 -> Gain/1
  Gain/1 -> ab0->abc/1

== system lib_dGrid/MMC-configurable control modes/MMC Control/CCSC + ZSCC control/PI regulator with anti-windup D ==
  note: Anti-windup mechanism: Method of conditionnal integration
      |
      | The integration is suspended if saturation occurs and the
      | control error is of the same sign as the control signal.
      |
      | [1] L.Rundqwist, "Anti-Reset Windup for PID Controllers," Ph.D. Thesis TRFT-1033,
      | Departement of Automatic Control, Lund Institute of Technology, Lund, Sweeden, 1991.
  Error : Inport  SampleTime=Ts
  Compare To Zero : simulink/Logic and Bit Operations/Compare To Zero  relop=>  OutDataTypeStr=uint8  ZeroCross=off
  Compare To Zero1 : simulink/Logic and Bit Operations/Compare To Zero  relop=<  OutDataTypeStr=uint8  ZeroCross=off
  Constant : Constant  Value=0
  Constant1 : Constant  Value=UpperLimit
  Constant3 : Constant  Value=LowerLimit
  Discrete-Time Integrator : DiscreteIntegrator  IntegratorMethod=Integration: Trapezoidal  InitialCondition=Init  SampleTime=Ts  LimitOutput=on  UpperSaturationLimit=UpperLimit  LowerSaturationLimit=LowerLimit  ShowStatePort=on  ICPrevOutput=DiscIntNeverNeededParam  ICPrevScaledInput=DiscIntNeverNeededParam
  Kp4 : Gain  Gain=Kp  SaturateOnIntegerOverflow=on  SampleTime=Ts  OutDataTypeStr=Inherit: Same as input  ParamDataTypeStr=Inherit: Same as input
  Kp5 : Gain  Gain=Ki  SaturateOnIntegerOverflow=on  SampleTime=Ts  OutDataTypeStr=Inherit: Same as input  ParamDataTypeStr=Inherit: Same as input
  Logical Operator : Logic  AllPortsSameDT=off  OutDataTypeStr=boolean
  Logical Operator1 : Logic  AllPortsSameDT=off  OutDataTypeStr=boolean
  Logical Operator2 : Logic  Operator=OR  AllPortsSameDT=off  OutDataTypeStr=boolean
  Relational Operator : RelationalOperator  OutDataTypeStr=boolean  InputSameDT=off
  Relational Operator1 : RelationalOperator  Operator=<=  OutDataTypeStr=boolean  InputSameDT=off
  Saturation2 : Saturate  UpperLimit=UpperLimit  LowerLimit=LowerLimit  SampleTime=Ts
  Sum1 : Sum  InputSameDT=on  SaturateOnIntegerOverflow=on  SampleTime=Ts  OutDataTypeStr=Inherit: Same as first input
  Sum6 : Sum  InputSameDT=on  SaturateOnIntegerOverflow=on  SampleTime=Ts  OutDataTypeStr=Inherit: Same as first input
  Switch : Switch  Criteria=u2 > Threshold  SaturateOnIntegerOverflow=off  InputSameDT=off
  Zero-Order Hold : ZeroOrderHold  SampleTime=Ts
  Out : Outport  SampleTime=Ts  InitialOutput=0  VectorParamsAs1DForOutWhenUnconnected=off
  wires:
  Constant/1 -> Switch/1
  Zero-Order Hold/1 -> Sum1/2, Sum6/1
  Discrete-Time Integrator/State -> Sum1/1
  Sum1/1 -> Relational Operator1/1, Relational Operator/1
  Logical Operator2/1 -> Switch/2
  Relational Operator/1 -> Logical Operator/1  "UpperLimit_is_Reached"
  Relational Operator1/1 -> Logical Operator1/1  "LowerLimit_Is_Reached"
  Constant1/1 -> Relational Operator/2
  Constant3/1 -> Relational Operator1/2
  Compare To Zero/1 -> Logical Operator/2  "Error_is_positive"
  Logical Operator/1 -> Logical Operator2/1
  Logical Operator1/1 -> Logical Operator2/2
  Compare To Zero1/1 -> Logical Operator1/2  "Error_is_negative"
  Error/1 -> Compare To Zero1/1, Compare To Zero/1, Kp4/1, Kp5/1
  Sum6/1 -> Saturation2/1
  Kp4/1 -> Zero-Order Hold/1
  Discrete-Time Integrator/1 -> Sum6/2
  Saturation2/1 -> Out/1
  Switch/1 -> Discrete-Time Integrator/1
  Kp5/1 -> Switch/3
